simulink model "controller_Arduino_ok"  (R2024b)
settings: Solver=FixedStepDiscrete  StartTime=0.0  StopTime=10  FixedStep=1/10  RelTol=1e-3
InitFcn:
  | init_fn()
libraries: arduinolib x17
settings Model: PacingRate=10  ExtModeTrigDuration=2  Creator=Jacopo Sini  LastModifiedBy=yoyom
settings SolverCC: AutoInsertRateTranBlk=on
settings OptimizationCC: EnhancedBackFolding=on  PassReuseOutputArgsAs=Individual arguments  ZeroExternalMemoryAtStartup=off  ZeroInternalMemoryAtStartup=off  MaxStackSize=64  OptimizeBlockOrder=speed  DifferentSizesBufferReuse=on  OptimizationCustomize=off  EfficientTunableParamExpr=on
settings DebuggingCC: ParameterTunabilityLossMsg=error  UnconnectedInputMsg=warning  UnconnectedOutputMsg=warning  UnconnectedLineMsg=warning
settings HardwareCC: ProdBitPerInt=16  ProdBitPerPointer=16  ProdBitPerSizeT=16  ProdBitPerPtrDiffT=16  ProdLargestAtomicFloat=None  ProdWordSize=8  ProdHWDeviceType=Atmel->AVR
settings SFSimCC: MATLABDynamicMemAlloc=off
settings RTWCC: Description=Embedded Coder  SystemTargetFile=ert.tlc  HardwareBoard=Arduino Uno  TemplateMakefile=ert_default_tmf  Toolchain=Arduino AVR  BuildConfiguration=Faster Runs  GPUComputeCapability=3.5  DLArmComputeVersion=19.05
settings CodeAppCC: ForceParamTrailComments=on  IgnoreCustomStorageClasses=off  OperatorAnnotations=on  SimulinkDataObjDesc=on  SFDataObjDesc=on  InsertBlockDesc=on
settings ERTTargetCC: SupportNonInlinedSFcns=on  SupportVariableSizeSignals=on  ExtModeTransport=3  ExtModeStaticAlloc=on  ExtModeAutomaticAllocSize=off  ExtModeStaticAllocSize=250  ExtModeMexFile=ext_xcp  ExtModeIntrfLevel=Level2 - Open  InlinedParameterPlacement=Hierarchical  ERTFilePackagingFormat=Compact
settings ConfigComp: CovMetricSettings=dcmwe

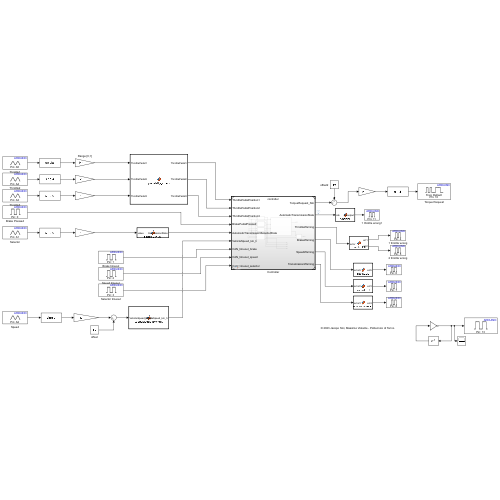
[thumbnail: Simulink's stored preview of the top-level diagram]
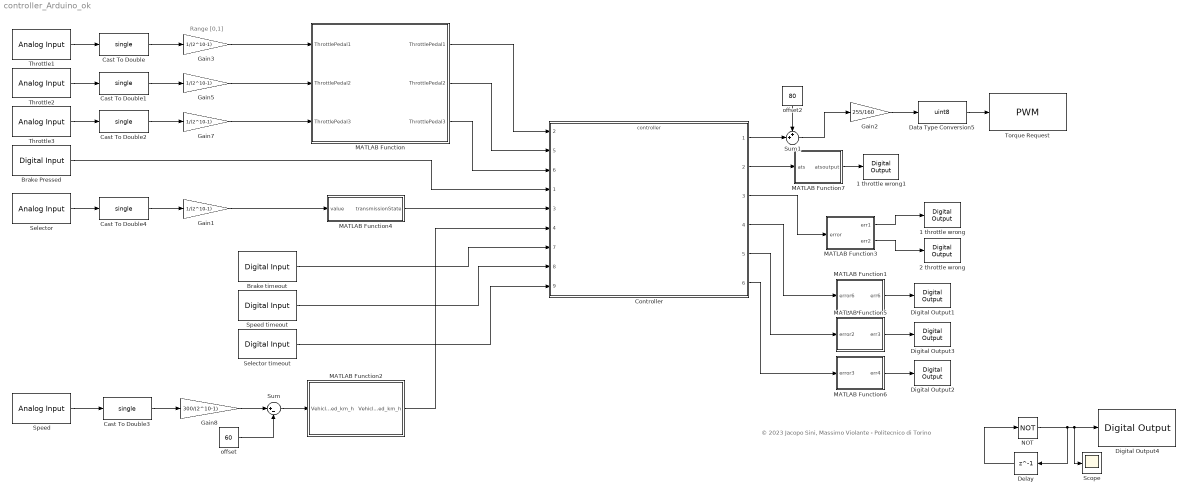
== system controller_Arduino_ok ==
  note: © 2023 Jacopo Sini, Massimo Violante - Politecnico di Torino
  note: Range [0,1]
  1 throttle wrong : arduinolib/Digital Output  pinNumber=4  Direction=output  blockPlatform=arduino
      settings: SourceProductName=Common
  1 throttle wrong1 : arduinolib/Digital Output  pinNumber=11  Direction=output  blockPlatform=arduino
      settings: SourceProductName=Common
  2 throttle wrong : arduinolib/Digital Output  pinNumber=5  Direction=output  blockPlatform=arduino
      settings: SourceProductName=Common
  Brake Pressed : arduinolib/Digital Input  pinNumber=0  mode=Default  Direction=input  SampleTime=0.1  blockPlatform=arduino
      settings: SourceProductName=Common
  Brake timeout : arduinolib/Digital Input  pinNumber=1  mode=Default  Direction=input  SampleTime=0.1  blockPlatform=arduino
      settings: SourceProductName=Common
  Cast To Double{,1..4} (5 alike) : DataTypeConversion  OutDataTypeStr=single  SaturateOnIntegerOverflow=off  RndMeth=Floor
  Controller : ModelReference  ModelNameDialog=controller  SimulationMode=Normal  ModelReferenceVersion=7.19
      settings: PortSchema="{\"entries\":[{\"content\":{\"sides\":[{\"content\":{\"connectorIds\":[\"In2\",\"In5\",\"In6\",\"In1\",\"In3\",\"In4\",\"In7\",\"In8\",\"In9\"]},\"type\":\"ConnectorPlacement.EquallySpacedRectSide\",\"uuid\":\"5e260b81-e1ce-497c-8572-ac5c2182ee27\"},{\"content\":{\"connectorIds\":[\"Out1\",\"Out2\",\"Out3\",\"Out4\",\"Out5\",\"Out6\"],\"side\":\"RIGHT\"},\"type\":\"ConnectorPlacement.EquallySpacedRectSide\",\"uuid\":\"4325f63c-e453-4c79-ab01-1476da99aa25\"},{\"content\":{\"side\":\"TOP\"},\"type\":\"ConnectorPlacement.EquallySpacedRectSide\",\"uuid\":\"dba88bac-0f95-4a98-ba3b-c40df5616f56\"}]},\"type\":\"ConnectorPlacement.EquallySpacedConnector\",\"uuid\":\"6943e10d-f3b0-4fd8-a142-b6b49e651f90\"}],\"packageUris\":[\"http://schema.mathworks.com/mf0/Connector/R2020b\"],\"version\":\"1.0\"}"
  Data Type Conversion5 : DataTypeConversion  OutDataTypeStr=uint8  SaturateOnIntegerOverflow=off  RndMeth=Floor
  Delay : Delay  DelayLength=1  SampleTime=0.5
  Digital Output1 : arduinolib/Digital Output  pinNumber=6  Direction=output  blockPlatform=arduino
      settings: SourceProductName=Common
  Digital Output2 : arduinolib/Digital Output  pinNumber=8  Direction=output  blockPlatform=arduino
      settings: SourceProductName=Common
  Digital Output3 : arduinolib/Digital Output  pinNumber=7  Direction=output  blockPlatform=arduino
      settings: SourceProductName=Common
  Digital Output4 : arduinolib/Digital Output  pinNumber=13  Direction=output  blockPlatform=arduino
      settings: SourceProductName=Common
  Gain{1,3,5,7} (4 alike) : Gain  Gain=1/(2^10-1)
  Gain2 : Gain  Gain=255/160
  Gain8 : Gain  Gain=300/(2^10-1)
  MATLAB Function : MATLAB Function  TreatAsAtomicUnit=on
  MATLAB Function1 : MATLAB Function  TreatAsAtomicUnit=on
  MATLAB Function2 : MATLAB Function  TreatAsAtomicUnit=on
  MATLAB Function3 : MATLAB Function  TreatAsAtomicUnit=on
  MATLAB Function4 : MATLAB Function  TreatAsAtomicUnit=on
  MATLAB Function5 : MATLAB Function  TreatAsAtomicUnit=on
  MATLAB Function6 : MATLAB Function  TreatAsAtomicUnit=on
  MATLAB Function7 : MATLAB Function  TreatAsAtomicUnit=on
  NOT : Logic  Operator=NOT  IconShape=distinctive  AllPortsSameDT=off  OutDataTypeStr=boolean
  Scope : Scope
  Selector : arduinolib/Analog Input  pinNumber=1  ReadResultsOnly=off  ConversionTriggerSource=Software  ExternalTriggerType=uint32( 0 )  OutputDataType=uint16  EnableConversionCompleteNotify=off  EnableOuputStatus=off  SampleTime=-1  blockPlatform=arduino
      settings: SourceProductName=Common
  Selector timeout : arduinolib/Digital Input  pinNumber=3  mode=Default  Direction=input  SampleTime=0.1  blockPlatform=arduino
      settings: SourceProductName=Common
  Speed : arduinolib/Analog Input  pinNumber=2  ReadResultsOnly=off  ConversionTriggerSource=Software  ExternalTriggerType=uint32( 0 )  OutputDataType=uint16  EnableConversionCompleteNotify=off  EnableOuputStatus=off  SampleTime=-1  blockPlatform=arduino
      settings: SourceProductName=Common
  Speed timeout : arduinolib/Digital Input  pinNumber=2  mode=Default  Direction=input  SampleTime=0.1  blockPlatform=arduino
      settings: SourceProductName=Common
  Sum : Sum  Inputs=|+-
  Sum1 : Sum  Inputs=++|
  Throttle1 : arduinolib/Analog Input  pinNumber=5  ReadResultsOnly=off  ConversionTriggerSource=Software  ExternalTriggerType=uint32( 0 )  OutputDataType=uint16  EnableConversionCompleteNotify=off  EnableOuputStatus=off  SampleTime=-1  blockPlatform=arduino
      settings: SourceProductName=Common
  Throttle2 : arduinolib/Analog Input  pinNumber=4  ReadResultsOnly=off  ConversionTriggerSource=Software  ExternalTriggerType=uint32( 0 )  OutputDataType=uint16  EnableConversionCompleteNotify=off  EnableOuputStatus=off  SampleTime=-1  blockPlatform=arduino
      settings: SourceProductName=Common
  Throttle3 : arduinolib/Analog Input  pinNumber=3  ReadResultsOnly=off  ConversionTriggerSource=Software  ExternalTriggerType=uint32( 0 )  OutputDataType=uint16  EnableConversionCompleteNotify=off  EnableOuputStatus=off  SampleTime=-1  blockPlatform=arduino
      settings: SourceProductName=Common
  Torque Request : arduinolib/PWM  pinNumber=10  frequencyType=Default  desiredFrequency=490.2  achievableFrequency=490.2
      settings: SourceProductName=Common
  offset : Constant  Value=60  OutDataTypeStr=single
  offset2 : Constant  Value=80
  wires:
  Controller/2 -> MATLAB Function7/1(ats)
  MATLAB Function/1(ThrottlePedal1) -> Controller/2
  MATLAB Function/2(ThrottlePedal2) -> Controller/5
  MATLAB Function/3(ThrottlePedal3) -> Controller/6
  Controller/3 -> MATLAB Function3/1(error)
  Controller/4 -> MATLAB Function1/1(error6)
  Controller/5 -> MATLAB Function5/1(error2)
  Controller/6 -> MATLAB Function6/1(error3)
  MATLAB Function3/2(err2) -> 2 throttle wrong/1
  MATLAB Function3/1(err1) -> 1 throttle wrong/1
  Throttle1/1 -> Cast To Double/1
  Cast To Double1/1 -> Gain5/1
  Cast To Double/1 -> Gain3/1
  Throttle2/1 -> Cast To Double1/1
  offset/1 -> Sum/2
  Cast To Double2/1 -> Gain7/1
  Throttle3/1 -> Cast To Double2/1
  Speed/1 -> Cast To Double3/1
  Cast To Double3/1 -> Gain8/1
  Gain3/1 -> MATLAB Function/1("ThrottlePedal1 ")
  Gain5/1 -> MATLAB Function/2("ThrottlePedal2 ")
  Gain7/1 -> MATLAB Function/3("ThrottlePedal3 ")
  Cast To Double4/1 -> Gain1/1
  Selector/1 -> Cast To Double4/1
  Gain1/1 -> MATLAB Function4/1(value)
  Brake Pressed/1 -> Controller/1
  Selector timeout/1 -> Controller/9
  Speed timeout/1 -> Controller/8
  Brake timeout/1 -> Controller/7
  MATLAB Function4/1(transmissionState) -> Controller/3
  MATLAB Function2/1(VehicleSpeed_km_h) -> Controller/4
  Gain8/1 -> Sum/1
  Sum/1 -> MATLAB Function2/1("VehicleSpeed_km_h ")
  Sum1/1 -> Gain2/1
  Controller/1 -> Sum1/2
  offset2/1 -> Sum1/1
  Gain2/1 -> Data Type Conversion5/1
  Data Type Conversion5/1 -> Torque Request/1
  Delay/1 -> NOT/1
  NOT/1 -> Delay/1, Scope/1, Digital Output4/1
  MATLAB Function1/1(err6) -> Digital Output1/1
  MATLAB Function6/1(err4) -> Digital Output2/1
  MATLAB Function5/1(err3) -> Digital Output3/1
  MATLAB Function7/1(atsoutput) -> 1 throttle wrong1/1

== matlab function controller_Arduino_ok/MATLAB Function2 ==
  data: VehicleSpeed_km_h output; VehicleSpeed_km_h input
function VehicleSpeed_km_h  = speedplausibilitycheck(VehicleSpeed_km_h)
    if(VehicleSpeed_km_h<-60 || VehicleSpeed_km_h>240) 
        VehicleSpeed_km_h=single(0);
    end

== matlab function controller_Arduino_ok/MATLAB Function1 ==
  data: err6 output boolean; error6 input single
function err6 = brakeLED(error6)
    err6 = false;
    if(error6>0)
        err6 = true;
    end

== matlab function controller_Arduino_ok/MATLAB Function3 ==
  data: err1 output boolean; error input single; err2 output boolean
function [err1, err2]= throttleLED(error)
    err1 = false;
    err2 = false;
    if(error>0)
        err1 = true;
    end
    if(error==2)
        err2 = true;
    end

== matlab function controller_Arduino_ok/MATLAB Function4 ==
  data: value input; transmissionState output
function transmissionState = double2enum(value)
    transmissionState = TransmissionState.Neutral;
    if(value>=0 && value<0.2)
        transmissionState = TransmissionState.Park;
    elseif(value>=0.2 && value<0.4)
        transmissionState = TransmissionState.Reverse;
    elseif(value>=0.4 && value<0.6)
        transmissionState = TransmissionState.Neutral;
    elseif(value>=0.6 && value<0.8)
        transmissionState = TransmissionState.Drive;
    elseif(value>=0.8 && value<=1)
        transmissionState = TransmissionState.Brake;
    end

== matlab function controller_Arduino_ok/MATLAB Function5 ==
  data: err3 output boolean; error2 input single
function err3 = speedLED(error2)
    err3 = false;
    if(error2>0)
        err3 = true;
    end

== matlab function controller_Arduino_ok/MATLAB Function6 ==
  data: err4 output boolean; error3 input single
function err4 = transmissionLED(error3)
    err4 = false;
    if(error3>0)
        err4 = true;
    end

== matlab function controller_Arduino_ok/MATLAB Function7 ==
  data: atsoutput output boolean; ats input
function atsoutput  = funzione(ats)
 atsoutput=false;
    if (ats==TransmissionState.Brake)
        atsoutput=true;
    end

== matlab function controller_Arduino_ok/MATLAB Function ==
  data: ThrottlePedal1 input; ThrottlePedal2 input; ThrottlePedal3 input; ThrottlePedal1 output; ThrottlePedal2 output; ThrottlePedal3 output
function [ThrottlePedal1,ThrottlePedal2,ThrottlePedal3]= plausibility_check(ThrottlePedal1,ThrottlePedal2,ThrottlePedal3)
    w1=single(0);
    w2=single(0);
    w3=single(0);
    if(ThrottlePedal1<0 || ThrottlePedal1>1) 
        ThrottlePedal1=single(-1);
        w1=single(1);
    end
    if(ThrottlePedal2<0 || ThrottlePedal2>1) 
        ThrottlePedal2=single(-3);
         w2=single(1);
    end
    if(ThrottlePedal3<0 || ThrottlePedal3>1) 
        ThrottlePedal3=single(-5);
         w3=single(1);
    end
